simulink model "fccr_balance"  (R2017b)
settings: Solver=FixedStepDiscrete  StartTime=0.0  StopTime=inf  RelTol=1e-3  EnableMultiTasking=on
undefined symbols (not defined in the file): DiscIntNeverNeededParam
libraries: beaglebonebluelib x6, simulink_extras x4, simulink x1
settings Model: SimulationMode=external  ExtModeTrigDuration=200  Creator=pthb3  LastModifiedBy=pthb3
settings SolverCC: PositivePriorityOrder=on
settings DataIOCC: InspectSignalLogs=on
settings OptimizationCC: PassReuseOutputArgsAs=Individual arguments  MaxStackSize=64
settings DebuggingCC: ParameterTunabilityLossMsg=error
settings HardwareCC: ProdBitPerPointer=32  ProdBitPerSizeT=32  ProdBitPerPtrDiffT=32  ProdLargestAtomicInteger=Long  ProdLargestAtomicFloat=Double  ProdWordSize=32  ProdHWDeviceType=ARM Compatible->ARM Cortex
settings SFSimCC: MATLABDynamicMemAlloc=off
settings RTWCC: SystemTargetFile=ert.tlc  HardwareBoard=Raspberry Pi  TemplateMakefile=ert_default_tmf  GenerateReport=on  Toolchain=GNU GCC Raspberry Pi  IncludeHyperlinkInReport=on  GenerateTraceInfo=on  GenerateTraceReport=on  GenerateTraceReportSl=on  GenerateTraceReportSf=on  GenerateTraceReportEml=on
settings CodeAppCC: ForceParamTrailComments=on  IgnoreCustomStorageClasses=off  OperatorAnnotations=on  SimulinkDataObjDesc=on  SFDataObjDesc=on  InsertBlockDesc=on
settings ERTTargetCC: SupportVariableSizeSignals=on

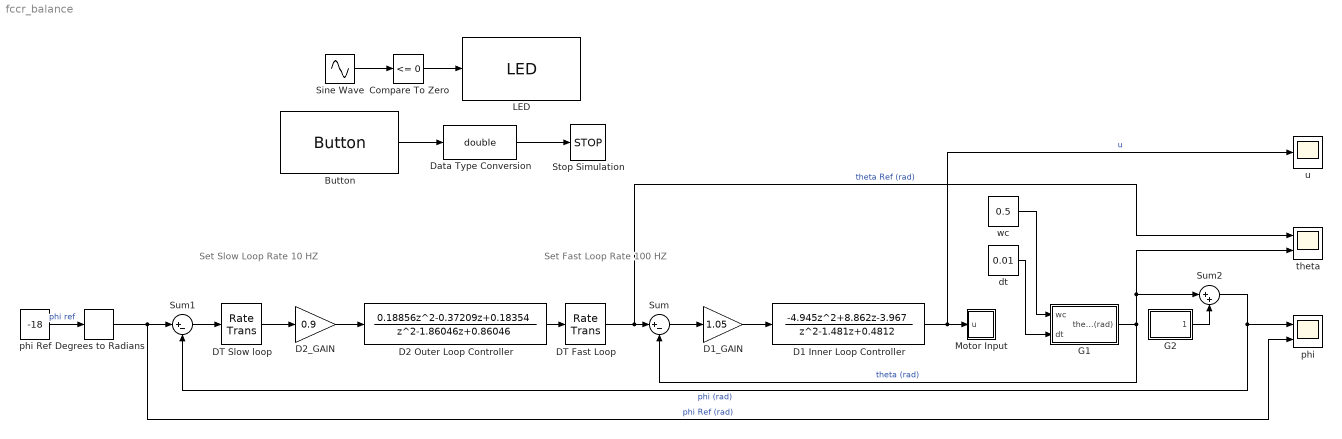
== system fccr_balance ==
  note: Set Slow Loop Rate
      | 10 HZ
  note: Set Fast Loop Rate
      | 100 HZ
  Button : beaglebonebluelib/Button  Button=Pause  SampleTime=0.1  SimulateUsing=Code generation
  Compare To Zero : simulink/Logic and Bit Operations/Compare To Zero  relop=<=  OutDataTypeStr=uint8
  D1 Inner Loop Controller : DiscreteTransferFcn  Numerator=[-4.945, 8.862, -3.967]  Denominator=[1.000, -1.481, 0.4812]
  D1_GAIN : Gain  Gain=1.05
  D2 Outer Loop Controller : DiscreteTransferFcn  Numerator="[0.18856,  -0.37209,  0.18354]"  Denominator="[1.00000,  -1.86046,   0.86046]"
  D2_GAIN : Gain  Gain=0.9
  DT Fast Loop : RateTransition  OutPortSampleTimeOpt=Multiple of input port sample time  OutPortSampleTimeMultiple=0.1  OutPortSampleTime=0.05
  DT Slow loop : RateTransition  OutPortSampleTime=0.1
  Data Type Conversion : DataTypeConversion  OutDataTypeStr=double
  Degrees to Radians : simulink_extras/Transformations/Degrees to Radians
  G1 : Subsystem
  G2 : Subsystem
  LED : beaglebonebluelib/LED  LED=Green
  Motor Input : Subsystem
  Sine Wave : Sin  SineType=Sample based  Frequency=3.14  SampleTime=0.1
  Stop Simulation : Stop
  Sum : Sum  Inputs=|+-
  Sum1 : Sum  Inputs=|+-
  Sum2 : Sum  Inputs=|++
  dt : Constant  Value=0.01
  phi : Scope  NumInputPorts=2
  phi Ref : Constant  Value=-18
  theta : Scope  NumInputPorts=2
  u : Scope
  wc : Constant  Value=0.5
  wires:
  Sine Wave/1 -> Compare To Zero/1
  Compare To Zero/1 -> LED/1
  D1_GAIN/1 -> D1 Inner Loop Controller/1
  D2_GAIN/1 -> D2 Outer Loop Controller/1
  Sum1/1 -> DT Slow loop/1
  Button/1 -> Data Type Conversion/1
  Data Type Conversion/1 -> Stop Simulation/1
  Sum/1 -> D1_GAIN/1
  G1/1(theta (rad)) -> Sum/2, theta/2, Sum2/1  "theta (rad)"
  wc/1 -> G1/1(wc)
  dt/1 -> G1/2(dt)
  DT Slow loop/1 -> D2_GAIN/1
  DT Fast Loop/1 -> theta/1, Sum/1  "theta Ref (rad)"
  phi Ref/1 -> Degrees to Radians/1  "phi ref"
  D1 Inner Loop Controller/1 -> Motor Input/1(u), u/1  "u"
  G2/1(phi (rad)) -> Sum2/2
  Sum2/1 -> phi/1, Sum1/2  "phi (rad)"
  Degrees to Radians/1 -> phi/2, Sum1/1  "phi Ref (rad)"
  D2 Outer Loop Controller/1 -> DT Fast Loop/1

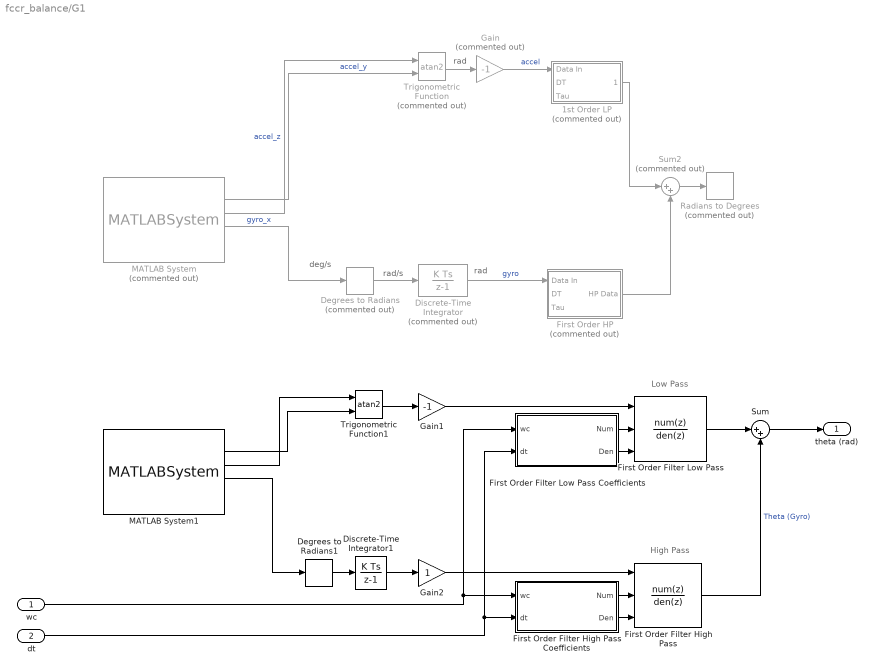
== system fccr_balance/G1 ==
  note: rad
  note: rad/s
  note: rad
  note: deg/s
  note: High Pass
  note: Low Pass
  wc : Inport
  dt : Inport  Port=2
  1st Order LP : Subsystem  Commented=on
  Degrees to Radians : simulink_extras/Transformations/Degrees to Radians  Commented=on
  Degrees to Radians1 : simulink_extras/Transformations/Degrees to Radians
  Discrete-Time Integrator : DiscreteIntegrator  Commented=on  InitialConditionSetting=State (most efficient)  SampleTime=-1  ICPrevOutput=DiscIntNeverNeededParam  ICPrevScaledInput=DiscIntNeverNeededParam
  Discrete-Time Integrator1 : DiscreteIntegrator  InitialConditionSetting=State (most efficient)  SampleTime=-1  ICPrevOutput=DiscIntNeverNeededParam  ICPrevScaledInput=DiscIntNeverNeededParam
  First Order Filter High Pass : DiscreteTransferFcn  NumeratorSource=Input port  DenominatorSource=Input port  Denominator=[1]  a0EqualsOne=on
      settings: InputPortMap=u0,p1,p3
  First Order Filter High Pass Coefficients : MATLAB Function  TreatAsAtomicUnit=on
  First Order Filter Low Pass : DiscreteTransferFcn  NumeratorSource=Input port  DenominatorSource=Input port  Denominator=[1]  a0EqualsOne=on
      settings: InputPortMap=u0,p1,p3
  First Order Filter Low Pass Coefficients : MATLAB Function  TreatAsAtomicUnit=on
  First Order HP : Subsystem  Commented=on
  Gain : Gain  Commented=on  Gain=-1
  Gain1 : Gain  Gain=-1
  Gain2 : Gain
  MATLAB System : MATLABSystem  Commented=on  System=beagleboneblue.fccr_bbblueIMU  SampleTime=0.01
      mask Type: beagleboneblue.fccr_bbblueIMU
      mask Display:
      | color('white');
      | plot([100,100,100,100]*1,[100,100,100,100]*1);
      | plot([100,100,100,100]*0,[100,100,100,100]*0);
      | color('blue');
      | text(100, 92, ' BB BLUE ', 'horizontalAlignment', 'right');
      | color('black');
      | text(52,52,' IMU','horizontalAlignment','center');
      | color('black');
  MATLAB System1 : MATLABSystem  System=beagleboneblue.fccr_bbblueIMU  SampleTime=0.01
      mask Type: beagleboneblue.fccr_bbblueIMU
      mask Display:
      | color('white');
      | plot([100,100,100,100]*1,[100,100,100,100]*1);
      | plot([100,100,100,100]*0,[100,100,100,100]*0);
      | color('blue');
      | text(100, 92, ' BB BLUE ', 'horizontalAlignment', 'right');
      | color('black');
      | text(52,52,' IMU','horizontalAlignment','center');
      | color('black');
  Radians to Degrees : simulink_extras/Transformations/Radians to Degrees  Commented=on
  Sum : Sum  Inputs=|++
  Sum2 : Sum  Commented=on  Inputs=|++
  Trigonometric Function : Trigonometry  Commented=on  Operator=atan2
  Trigonometric Function1 : Trigonometry  Operator=atan2
  theta (rad) : Outport
  wires:
  MATLAB System/2 -> Trigonometric Function/2  "accel_y"
  MATLAB System/3 -> Trigonometric Function/1  "accel_z"
  MATLAB System/4 -> Degrees to Radians/1  "gyro_x"
  Discrete-Time Integrator/1 -> First Order HP/1(Data In)  "gyro"
  Degrees to Radians/1 -> Discrete-Time Integrator/1
  Trigonometric Function/1 -> Gain/1
  1st Order LP/1(LP Data) -> Sum2/1
  Sum2/1 -> Radians to Degrees/1
  Gain/1 -> 1st Order LP/1(Data In)  "accel"
  First Order HP/1(HP Data) -> Sum2/2
  First Order Filter Low Pass Coefficients/1(Num) -> First Order Filter Low Pass/2
  Gain2/1 -> First Order Filter High Pass/1
  First Order Filter Low Pass Coefficients/2(Den) -> First Order Filter Low Pass/3
  MATLAB System1/4 -> Degrees to Radians1/1
  Trigonometric Function1/1 -> Gain1/1
  wc/1 -> First Order Filter Low Pass Coefficients/1(wc), First Order Filter High Pass Coefficients/1(wc)
  dt/1 -> First Order Filter Low Pass Coefficients/2(dt), First Order Filter High Pass Coefficients/2(dt)
  First Order Filter High Pass Coefficients/2(Den) -> First Order Filter High Pass/3
  First Order Filter Low Pass/1 -> Sum/1
  Gain1/1 -> First Order Filter Low Pass/1
  Discrete-Time Integrator1/1 -> Gain2/1
  First Order Filter High Pass/1 -> Sum/2  "Theta (Gyro)"
  Degrees to Radians1/1 -> Discrete-Time Integrator1/1
  Sum/1 -> theta (rad)/1
  MATLAB System1/2 -> Trigonometric Function1/2
  First Order Filter High Pass Coefficients/1(Num) -> First Order Filter High Pass/2
  MATLAB System1/3 -> Trigonometric Function1/1

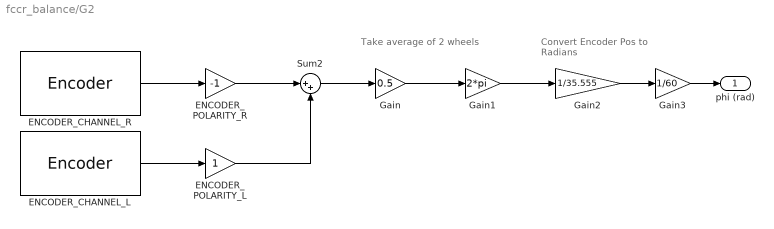
== system fccr_balance/G2 ==
  note: Convert Encoder Pos
      | to Radians
  note: Take average
      | of 2 wheels
  ENCODER_CHANNEL_L : beaglebonebluelib/Encoder  Channel=3  Mode=No reset  SampleTime=0.01  SimulateUsing=Code generation
  ENCODER_CHANNEL_R : beaglebonebluelib/Encoder  Channel=2  Mode=No reset  SampleTime=0.01  SimulateUsing=Code generation
  ENCODER_POLARITY_L : Gain
  ENCODER_POLARITY_R : Gain  Gain=-1
  Gain : Gain  Gain=0.5  OutDataTypeStr=double
  Gain1 : Gain  Gain=2*pi
  Gain2 : Gain  Gain=1/35.555
  Gain3 : Gain  Gain=1/60
  Sum2 : Sum  Inputs=|++
  phi (rad) : Outport
  wires:
  ENCODER_POLARITY_R/1 -> Sum2/1
  ENCODER_POLARITY_L/1 -> Sum2/2
  ENCODER_CHANNEL_L/1 -> ENCODER_POLARITY_L/1
  ENCODER_CHANNEL_R/1 -> ENCODER_POLARITY_R/1
  Sum2/1 -> Gain/1
  Gain/1 -> Gain1/1
  Gain1/1 -> Gain2/1
  Gain2/1 -> Gain3/1
  Gain3/1 -> phi (rad)/1

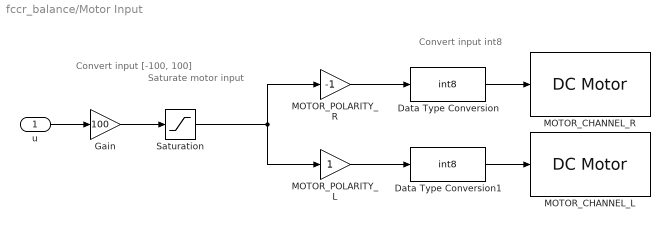
== system fccr_balance/Motor Input ==
  note: Saturate motor
      | input
  note: Convert input
      | int8
  note: Convert input
      | [-100, 100]
  u : Inport
  Data Type Conversion : DataTypeConversion  OutDataTypeStr=int8  SaturateOnIntegerOverflow=on  RndMeth=Zero
  Data Type Conversion1 : DataTypeConversion  OutDataTypeStr=int8  SaturateOnIntegerOverflow=on  RndMeth=Zero
  Gain : Gain  Gain=100
  MOTOR_CHANNEL_L : beaglebonebluelib/DC Motor  index=3  stopaction=Free Spin  SimulateUsing=Code generation
  MOTOR_CHANNEL_R : beaglebonebluelib/DC Motor  index=2  stopaction=Free Spin  SimulateUsing=Code generation
  MOTOR_POLARITY_L : Gain
  MOTOR_POLARITY_R : Gain  Gain=-1
  Saturation : Saturate  UpperLimit=100  LowerLimit=-100
  wires:
  u/1 -> Gain/1
  Gain/1 -> Saturation/1
  MOTOR_POLARITY_R/1 -> Data Type Conversion/1
  MOTOR_POLARITY_L/1 -> Data Type Conversion1/1
  Saturation/1 -> MOTOR_POLARITY_R/1, MOTOR_POLARITY_L/1
  Data Type Conversion/1 -> MOTOR_CHANNEL_R/1
  Data Type Conversion1/1 -> MOTOR_CHANNEL_L/1

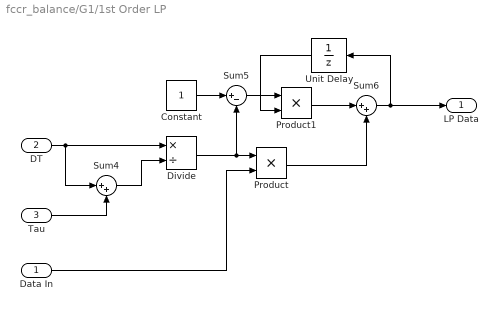
== system fccr_balance/G1/1st Order LP ==
  Data In : Inport
  DT : Inport  Port=2
  Tau : Inport  Port=3
  Constant : Constant
  Divide : Product  Inputs=*/
  Product : Product
  Product1 : Product
  Sum4 : Sum  Inputs=|++
  Sum5 : Sum  Inputs=|+-
  Sum6 : Sum  Inputs=|++
  Unit Delay : UnitDelay  SampleTime=-1
  LP Data : Outport
  wires:
  DT/1 -> Sum4/1, Divide/1
  Sum5/1 -> Product1/1
  Product/1 -> Sum6/2
  Tau/1 -> Sum4/2
  Divide/1 -> Product/1, Sum5/2
  Constant/1 -> Sum5/1
  Data In/1 -> Product/2
  Product1/1 -> Sum6/1
  Sum4/1 -> Divide/2
  Sum6/1 -> LP Data/1, Unit Delay/1
  Unit Delay/1 -> Product1/2

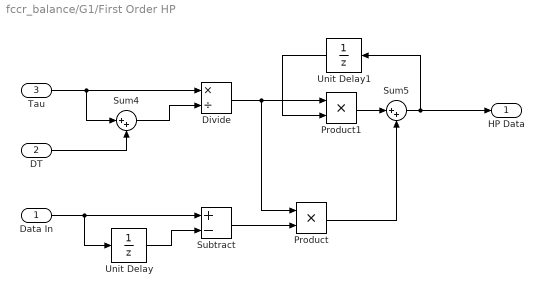
== system fccr_balance/G1/First Order HP ==
  Data In : Inport
  DT : Inport  Port=2
  Tau : Inport  Port=3
  Divide : Product  Inputs=*/
  Product : Product
  Product1 : Product
  Subtract : Sum  Inputs=+-
  Sum4 : Sum  Inputs=|++
  Sum5 : Sum  Inputs=|++
  Unit Delay : UnitDelay  SampleTime=-1
  Unit Delay1 : UnitDelay  SampleTime=-1
  HP Data : Outport
  wires:
  Subtract/1 -> Product/2
  Divide/1 -> Product1/1, Product/1
  Data In/1 -> Unit Delay/1, Subtract/1
  Tau/1 -> Divide/1, Sum4/1
  DT/1 -> Sum4/2
  Product/1 -> Sum5/2
  Sum5/1 -> HP Data/1, Unit Delay1/1
  Sum4/1 -> Divide/2
  Unit Delay/1 -> Subtract/2
  Product1/1 -> Sum5/1
  Unit Delay1/1 -> Product1/2

== matlab function fccr_balance/G1/First Order Filter High Pass Coefficients ==
  data: wc input; Num output; dt input; Den output
function [Num, Den] = first_order_hp(wc,dt)
%#codegen
Num = [1 -1];
Den = [1 (wc*dt - 1)];

== matlab function fccr_balance/G1/First Order Filter Low Pass Coefficients ==
  data: wc input; Num output; dt input; Den output
function [Num, Den] = first_order_lp(wc,dt)
%#codegen
Num = [0 wc*dt];
Den = [1 (wc*dt - 1)];
